simulink model "MdEnChk4s"  (R2018b)
settings: Solver=FixedStepDiscrete  StartTime=0.0  StopTime=10.0  FixedStep=0.01  RelTol=1e-3
undefined symbols (not defined in the file or in its folder): ChkBsyBit, MdAvl, MdEnChk_MdXX_Cal, Req, SetBsyBit, SetEnBit
settings Model: Creator=sn2xws  LastModifiedBy=sn2xws
settings DataIOCC: SaveFormat=StructureWithTime
settings OptimizationCC: DefaultParameterBehavior=Inlined  EnhancedBackFolding=on  PassReuseOutputArgsAs=Individual arguments  ZeroExternalMemoryAtStartup=off  ZeroInternalMemoryAtStartup=off  OptimizeBlockOrder=speed  DifferentSizesBufferReuse=on  OptimizationCustomize=off
settings DebuggingCC: ParameterTunabilityLossMsg=error
settings ModelReferenceCC: ModelReferenceNumInstancesAllowed=Single
settings SFSimCC: MATLABDynamicMemAlloc=off
settings RTWCC: SystemTargetFile=autosar.tlc  GenCodeOnly=on  TemplateMakefile=ert_default_tmf  Description=AUTOSAR  GenerateReport=on  IncludeHyperlinkInReport=on  LaunchReport=on  GenerateTraceInfo=on  GenerateTraceReport=on  GenerateTraceReportSl=on  GenerateTraceReportSf=on  GenerateTraceReportEml=on  GenerateCodeMetricsReport=on
settings CodeAppCC: ForceParamTrailComments=on  IgnoreCustomStorageClasses=off  OperatorAnnotations=on  SimulinkDataObjDesc=on  SFDataObjDesc=on  InsertBlockDesc=on
settings STFCustomTargetCC: TargetLangStandard=C99 (ISO)  MultiwordLength=256  ParMdlRefBuildCompliant=on  CompOptLevelCompliant=on  IncludeMdlTerminateFcn=off  CombineOutputUpdateFcns=on  SuppressErrorStatus=on  ERTCustomFileBanners=on  SupportNonFinite=off  SupportComplex=off  SupportContinuousTime=off  SupportNonInlinedSFcns=off  RemoveResetFunc=on  MATLABClassNameForMDSCustomization=Simulink.SoftwareTarget.ERTCustomization  AutosarCompliant=on  UseToolchainInfoCompliant=on  LookupTableObjectStructAxisOrder=2,1,3,4,...  LUTObjectStructOrderEvenSpacing=Size,Table,Breakpoints  SystemTargetFile=autosar.tlc
settings ERTTargetCC: TargetLangStandard=C99 (ISO)  ConcurrentExecutionCompliant=off  IncludeMdlTerminateFcn=off  SuppressErrorStatus=on  SupportNonFinite=off  SupportComplex=off  ModelStepFunctionPrototypeControlCompliant=off  CPPClassGenCompliant=off  AutosarCompliant=on  LookupTableObjectStructAxisOrder=2,1,3,4,...  LUTObjectStructOrderEvenSpacing=Size,Table,Breakpoints  InlinedParameterPlacement=NonHierarchical  ERTCustomFileTemplate=example_file_process.tlc  ERTFilePackagingFormat=Compact

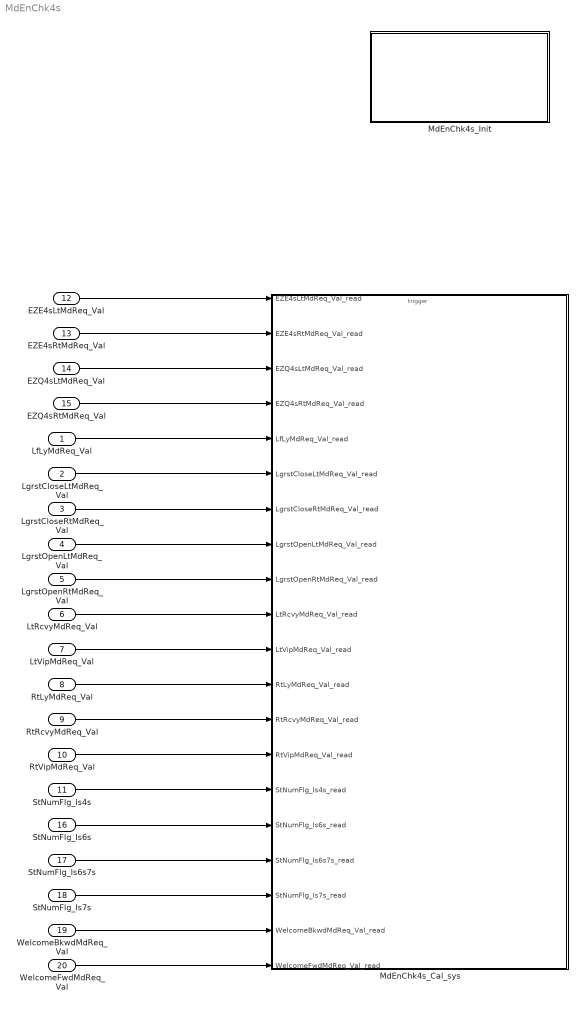
== system MdEnChk4s ==
  LfLyMdReq_Val : Inport  OutDataTypeStr=boolean  PortDimensions=1
  LgrstCloseLtMdReq_Val : Inport  Port=2  OutDataTypeStr=boolean  PortDimensions=1
  LgrstCloseRtMdReq_Val : Inport  Port=3  OutDataTypeStr=boolean  PortDimensions=1
  LgrstOpenLtMdReq_Val : Inport  Port=4  OutDataTypeStr=boolean  PortDimensions=1
  LgrstOpenRtMdReq_Val : Inport  Port=5  OutDataTypeStr=boolean  PortDimensions=1
  LtRcvyMdReq_Val : Inport  Port=6  OutDataTypeStr=boolean  PortDimensions=1
  LtVipMdReq_Val : Inport  Port=7  OutDataTypeStr=boolean  PortDimensions=1
  RtLyMdReq_Val : Inport  Port=8  OutDataTypeStr=boolean  PortDimensions=1
  RtRcvyMdReq_Val : Inport  Port=9  OutDataTypeStr=boolean  PortDimensions=1
  RtVipMdReq_Val : Inport  Port=10  OutDataTypeStr=boolean  PortDimensions=1
  StNumFlg_Is4s : Inport  Port=11  OutDataTypeStr=boolean  PortDimensions=1
  EZE4sLtMdReq_Val : Inport  Port=12  OutDataTypeStr=boolean  PortDimensions=1
  EZE4sRtMdReq_Val : Inport  Port=13  OutDataTypeStr=boolean  PortDimensions=1
  EZQ4sLtMdReq_Val : Inport  Port=14  OutDataTypeStr=boolean  PortDimensions=1
  EZQ4sRtMdReq_Val : Inport  Port=15  OutDataTypeStr=boolean  PortDimensions=1
  StNumFlg_Is6s : Inport  Port=16  OutDataTypeStr=boolean  PortDimensions=1
  StNumFlg_Is6s7s : Inport  Port=17  OutDataTypeStr=boolean  PortDimensions=1
  StNumFlg_Is7s : Inport  Port=18  OutDataTypeStr=boolean  PortDimensions=1
  WelcomeBkwdMdReq_Val : Inport  Port=19  OutDataTypeStr=boolean  PortDimensions=1
  WelcomeFwdMdReq_Val : Inport  Port=20  OutDataTypeStr=boolean  PortDimensions=1
  MdEnChk4s_Cal_sys : Subsystem
  MdEnChk4s_Init : Subsystem
  wires:
  LfLyMdReq_Val/1 -> MdEnChk4s_Cal_sys/5(LfLyMdReq_Val_read)
  LgrstCloseLtMdReq_Val/1 -> MdEnChk4s_Cal_sys/6(LgrstCloseLtMdReq_Val_read)
  LgrstCloseRtMdReq_Val/1 -> MdEnChk4s_Cal_sys/7(LgrstCloseRtMdReq_Val_read)
  LgrstOpenLtMdReq_Val/1 -> MdEnChk4s_Cal_sys/8(LgrstOpenLtMdReq_Val_read)
  LgrstOpenRtMdReq_Val/1 -> MdEnChk4s_Cal_sys/9(LgrstOpenRtMdReq_Val_read)
  LtRcvyMdReq_Val/1 -> MdEnChk4s_Cal_sys/10(LtRcvyMdReq_Val_read)
  LtVipMdReq_Val/1 -> MdEnChk4s_Cal_sys/11(LtVipMdReq_Val_read)
  RtLyMdReq_Val/1 -> MdEnChk4s_Cal_sys/12(RtLyMdReq_Val_read)
  RtRcvyMdReq_Val/1 -> MdEnChk4s_Cal_sys/13(RtRcvyMdReq_Val_read)
  RtVipMdReq_Val/1 -> MdEnChk4s_Cal_sys/14(RtVipMdReq_Val_read)
  StNumFlg_Is4s/1 -> MdEnChk4s_Cal_sys/15(StNumFlg_Is4s_read)
  EZE4sLtMdReq_Val/1 -> MdEnChk4s_Cal_sys/1(EZE4sLtMdReq_Val_read)
  EZE4sRtMdReq_Val/1 -> MdEnChk4s_Cal_sys/2(EZE4sRtMdReq_Val_read)
  EZQ4sLtMdReq_Val/1 -> MdEnChk4s_Cal_sys/3(EZQ4sLtMdReq_Val_read)
  EZQ4sRtMdReq_Val/1 -> MdEnChk4s_Cal_sys/4(EZQ4sRtMdReq_Val_read)
  StNumFlg_Is6s/1 -> MdEnChk4s_Cal_sys/16(StNumFlg_Is6s_read)
  StNumFlg_Is6s7s/1 -> MdEnChk4s_Cal_sys/17(StNumFlg_Is6s7s_read)
  StNumFlg_Is7s/1 -> MdEnChk4s_Cal_sys/18(StNumFlg_Is7s_read)
  WelcomeBkwdMdReq_Val/1 -> MdEnChk4s_Cal_sys/19(WelcomeBkwdMdReq_Val_read)
  WelcomeFwdMdReq_Val/1 -> MdEnChk4s_Cal_sys/20(WelcomeFwdMdReq_Val_read)

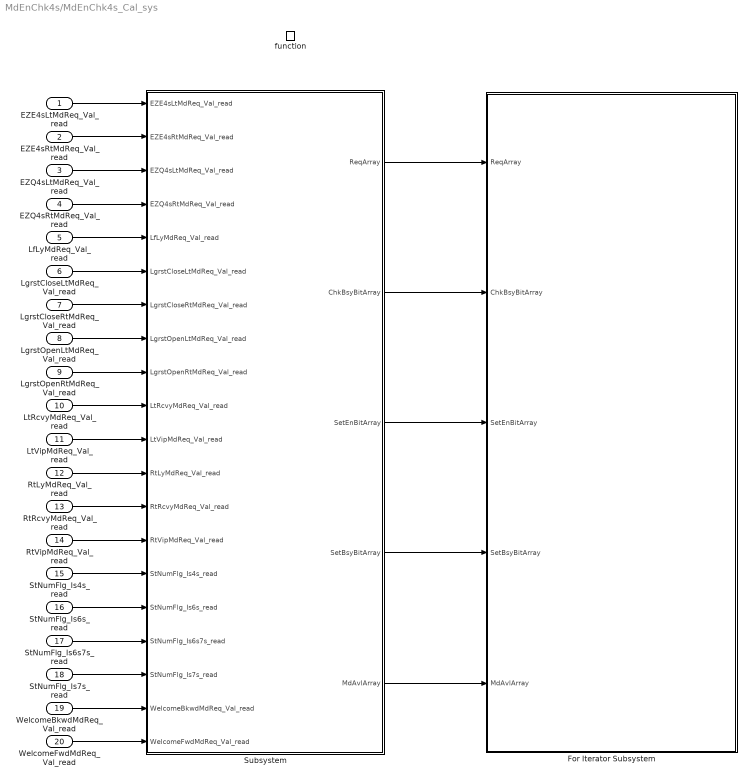
== system MdEnChk4s/MdEnChk4s_Cal_sys ==
  EZE4sLtMdReq_Val_read : Inport
  EZE4sRtMdReq_Val_read : Inport  Port=2
  EZQ4sLtMdReq_Val_read : Inport  Port=3
  EZQ4sRtMdReq_Val_read : Inport  Port=4
  LfLyMdReq_Val_read : Inport  Port=5
  LgrstCloseLtMdReq_Val_read : Inport  Port=6
  LgrstCloseRtMdReq_Val_read : Inport  Port=7
  LgrstOpenLtMdReq_Val_read : Inport  Port=8
  LgrstOpenRtMdReq_Val_read : Inport  Port=9
  LtRcvyMdReq_Val_read : Inport  Port=10
  LtVipMdReq_Val_read : Inport  Port=11
  RtLyMdReq_Val_read : Inport  Port=12
  RtRcvyMdReq_Val_read : Inport  Port=13
  RtVipMdReq_Val_read : Inport  Port=14
  StNumFlg_Is4s_read : Inport  Port=15
  StNumFlg_Is6s_read : Inport  Port=16
  StNumFlg_Is6s7s_read : Inport  Port=17
  StNumFlg_Is7s_read : Inport  Port=18
  WelcomeBkwdMdReq_Val_read : Inport  Port=19
  WelcomeFwdMdReq_Val_read : Inport  Port=20
  function : TriggerPort  TriggerType=function-call  IsSimulinkFunction=on  FunctionName=MdEnChk4s_Cal  VariantControl=(inherit)
  For Iterator Subsystem : Subsystem  TreatAsAtomicUnit=on
  Subsystem : Subsystem
  wires:
  EZE4sLtMdReq_Val_read/1 -> Subsystem/1(EZE4sLtMdReq_Val_read)
  EZE4sRtMdReq_Val_read/1 -> Subsystem/2(EZE4sRtMdReq_Val_read)
  EZQ4sLtMdReq_Val_read/1 -> Subsystem/3(EZQ4sLtMdReq_Val_read)
  EZQ4sRtMdReq_Val_read/1 -> Subsystem/4(EZQ4sRtMdReq_Val_read)
  LfLyMdReq_Val_read/1 -> Subsystem/5(LfLyMdReq_Val_read)
  LgrstCloseLtMdReq_Val_read/1 -> Subsystem/6(LgrstCloseLtMdReq_Val_read)
  LgrstCloseRtMdReq_Val_read/1 -> Subsystem/7(LgrstCloseRtMdReq_Val_read)
  LgrstOpenLtMdReq_Val_read/1 -> Subsystem/8(LgrstOpenLtMdReq_Val_read)
  LgrstOpenRtMdReq_Val_read/1 -> Subsystem/9(LgrstOpenRtMdReq_Val_read)
  LtRcvyMdReq_Val_read/1 -> Subsystem/10(LtRcvyMdReq_Val_read)
  LtVipMdReq_Val_read/1 -> Subsystem/11(LtVipMdReq_Val_read)
  RtLyMdReq_Val_read/1 -> Subsystem/12(RtLyMdReq_Val_read)
  RtRcvyMdReq_Val_read/1 -> Subsystem/13(RtRcvyMdReq_Val_read)
  RtVipMdReq_Val_read/1 -> Subsystem/14(RtVipMdReq_Val_read)
  StNumFlg_Is4s_read/1 -> Subsystem/15(StNumFlg_Is4s_read)
  StNumFlg_Is6s_read/1 -> Subsystem/16(StNumFlg_Is6s_read)
  StNumFlg_Is6s7s_read/1 -> Subsystem/17(StNumFlg_Is6s7s_read)
  StNumFlg_Is7s_read/1 -> Subsystem/18(StNumFlg_Is7s_read)
  WelcomeBkwdMdReq_Val_read/1 -> Subsystem/19(WelcomeBkwdMdReq_Val_read)
  WelcomeFwdMdReq_Val_read/1 -> Subsystem/20(WelcomeFwdMdReq_Val_read)
  Subsystem/1(ReqArray) -> For Iterator Subsystem/1(ReqArray)
  Subsystem/2(ChkBsyBitArray) -> For Iterator Subsystem/2(ChkBsyBitArray)
  Subsystem/3(SetEnBitArray) -> For Iterator Subsystem/3(SetEnBitArray)
  Subsystem/4(SetBsyBitArray) -> For Iterator Subsystem/4(SetBsyBitArray)
  Subsystem/5(MdAvlArray) -> For Iterator Subsystem/5(MdAvlArray)

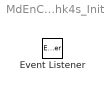
== system MdEnChk4s/MdEnChk4s_Init ==
  Event Listener : EventListener  EventName=reset

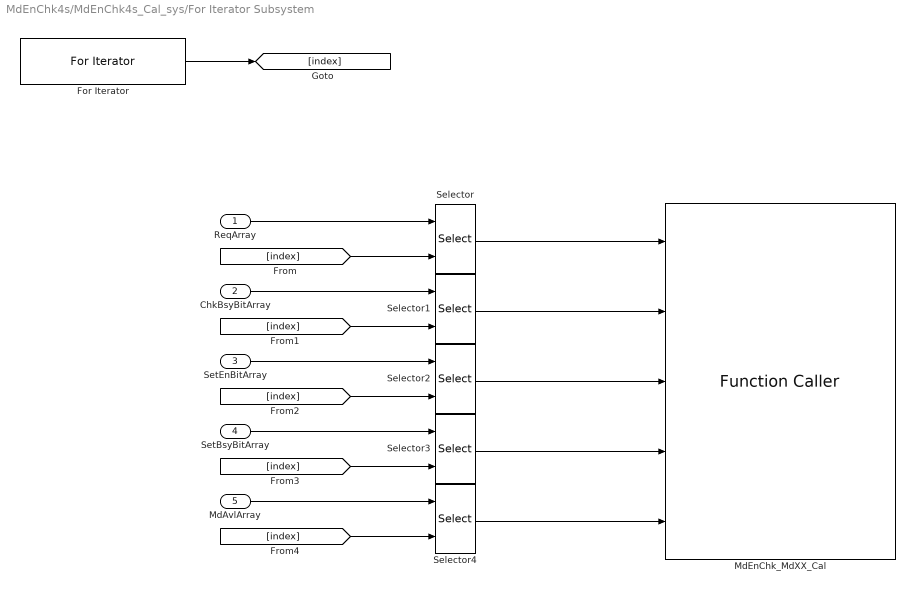
== system MdEnChk4s/MdEnChk4s_Cal_sys/For Iterator Subsystem ==
  ReqArray : Inport
  ChkBsyBitArray : Inport  Port=2
  SetEnBitArray : Inport  Port=3
  SetBsyBitArray : Inport  Port=4
  MdAvlArray : Inport  Port=5
  For Iterator : ForIterator  IterationLimit=16  IndexMode=Zero-based  IterationVariableDataType=int8
  MdEnChk_MdXX_Cal : FunctionCaller  Description=|  FunctionPrototype=MdEnChk_MdXX_Cal(Req,ChkBsyBit,SetEnBit,SetBsyBit,MdAvl)  InputArgumentSpecifications=boolean(true), uint32(1), uint32(1), uint32(1), boolean(true)
      | StNun: 
      | 0 :4s
      | 1:6s
      | 2:7s
      | 3:4sp
  Selector{,1..4} (5 alike) : Selector  IndexMode=Zero-based  InputPortWidth=16  IndexOptions=Index vector (port)  Indices=[1 3]  OutputSizes=1
  wires:
  For Iterator/1 -> [index]
  [index] -> Selector/2
  Selector/1 -> MdEnChk_MdXX_Cal/1
  ReqArray/1 -> Selector/1
  ChkBsyBitArray/1 -> Selector1/1
  [index] -> Selector1/2
  Selector1/1 -> MdEnChk_MdXX_Cal/2
  [index] -> Selector2/2
  SetEnBitArray/1 -> Selector2/1
  Selector2/1 -> MdEnChk_MdXX_Cal/3
  SetBsyBitArray/1 -> Selector3/1
  [index] -> Selector3/2
  Selector3/1 -> MdEnChk_MdXX_Cal/4
  Selector4/1 -> MdEnChk_MdXX_Cal/5
  [index] -> Selector4/2
  MdAvlArray/1 -> Selector4/1

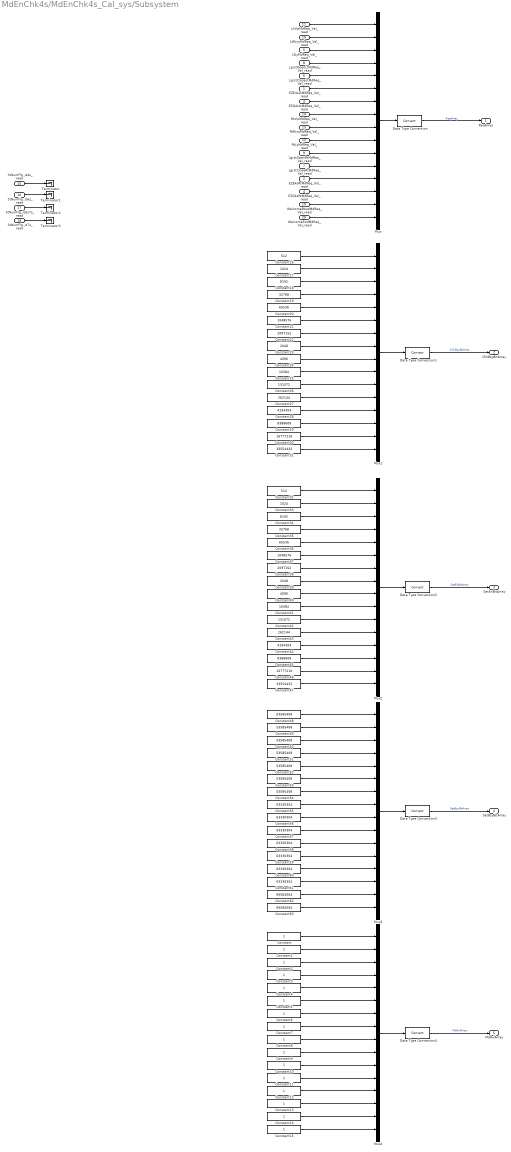
== system MdEnChk4s/MdEnChk4s_Cal_sys/Subsystem ==
  EZE4sLtMdReq_Val_read : Inport
  EZE4sRtMdReq_Val_read : Inport  Port=2
  EZQ4sLtMdReq_Val_read : Inport  Port=3
  EZQ4sRtMdReq_Val_read : Inport  Port=4
  LfLyMdReq_Val_read : Inport  Port=5
  LgrstCloseLtMdReq_Val_read : Inport  Port=6
  LgrstCloseRtMdReq_Val_read : Inport  Port=7
  LgrstOpenLtMdReq_Val_read : Inport  Port=8
  LgrstOpenRtMdReq_Val_read : Inport  Port=9
  LtRcvyMdReq_Val_read : Inport  Port=10
  LtVipMdReq_Val_read : Inport  Port=11
  RtLyMdReq_Val_read : Inport  Port=12
  RtRcvyMdReq_Val_read : Inport  Port=13
  RtVipMdReq_Val_read : Inport  Port=14
  StNumFlg_Is4s_read : Inport  Port=15
  StNumFlg_Is6s_read : Inport  Port=16
  StNumFlg_Is6s7s_read : Inport  Port=17
  StNumFlg_Is7s_read : Inport  Port=18
  WelcomeBkwdMdReq_Val_read : Inport  Port=19
  WelcomeFwdMdReq_Val_read : Inport  Port=20
  Constant{,1..15} (16 alike) : Constant  OutDataTypeStr=boolean
  Constant16 : Constant  Value=512  OutDataTypeStr=uint32
  Constant17 : Constant  Value=1024  OutDataTypeStr=uint32
  Constant18 : Constant  Value=8192  OutDataTypeStr=uint32
  Constant19 : Constant  Value=32768  OutDataTypeStr=uint32
  Constant20 : Constant  Value=65536  OutDataTypeStr=uint32
  Constant21 : Constant  Value=1048576  OutDataTypeStr=uint32
  Constant22 : Constant  Value=2097152  OutDataTypeStr=uint32
  Constant23 : Constant  Value=2048  OutDataTypeStr=uint32
  Constant24 : Constant  Value=4096  OutDataTypeStr=uint32
  Constant25 : Constant  Value=16384  OutDataTypeStr=uint32
  Constant26 : Constant  Value=131072  OutDataTypeStr=uint32
  Constant27 : Constant  Value=262144  OutDataTypeStr=uint32
  Constant28 : Constant  Value=4194304  OutDataTypeStr=uint32
  Constant29 : Constant  Value=8388608  OutDataTypeStr=uint32
  Constant30 : Constant  Value=16777216  OutDataTypeStr=uint32
  Constant31 : Constant  Value=33554432  OutDataTypeStr=uint32
  Constant32 : Constant  Value=512  OutDataTypeStr=uint32
  Constant33 : Constant  Value=1024  OutDataTypeStr=uint32
  Constant34 : Constant  Value=8192  OutDataTypeStr=uint32
  Constant35 : Constant  Value=32768  OutDataTypeStr=uint32
  Constant36 : Constant  Value=65536  OutDataTypeStr=uint32
  Constant37 : Constant  Value=1048576  OutDataTypeStr=uint32
  Constant38 : Constant  Value=2097152  OutDataTypeStr=uint32
  Constant39 : Constant  Value=2048  OutDataTypeStr=uint32
  Constant40 : Constant  Value=4096  OutDataTypeStr=uint32
  Constant41 : Constant  Value=16384  OutDataTypeStr=uint32
  Constant42 : Constant  Value=131072  OutDataTypeStr=uint32
  Constant43 : Constant  Value=262144  OutDataTypeStr=uint32
  Constant44 : Constant  Value=4194304  OutDataTypeStr=uint32
  Constant45 : Constant  Value=8388608  OutDataTypeStr=uint32
  Constant46 : Constant  Value=16777216  OutDataTypeStr=uint32
  Constant47 : Constant  Value=33554432  OutDataTypeStr=uint32
  Constant{48..54} (7 alike) : Constant  Value=53585408  OutDataTypeStr=uint32
  Constant{55..61} (7 alike) : Constant  Value=63330304  OutDataTypeStr=uint32
  Constant62 : Constant  Value=66584064  OutDataTypeStr=uint32
  Constant63 : Constant  Value=66584064  OutDataTypeStr=uint32
  Data Type Conversion{,1..4} (5 alike) : DataTypeConversion
  Mux{,1..4} (5 alike) : Mux  Inputs=16
  Terminator{,1..3} (4 alike) : Terminator
  ReqArray : Outport
  ChkBsyBitArray : Outport  Port=2
  SetEnBitArray : Outport  Port=3
  SetBsyBitArray : Outport  Port=4
  MdAvlArray : Outport  Port=5
  wires:
  LgrstOpenLtMdReq_Val_read/1 -> Mux/4
  LgrstCloseLtMdReq_Val_read/1 -> Mux/5
  EZE4sLtMdReq_Val_read/1 -> Mux/6
  RtRcvyMdReq_Val_read/1 -> Mux/9
  RtLyMdReq_Val_read/1 -> Mux/10
  LgrstOpenRtMdReq_Val_read/1 -> Mux/11
  LgrstCloseRtMdReq_Val_read/1 -> Mux/12
  LtVipMdReq_Val_read/1 -> Mux/1
  LtRcvyMdReq_Val_read/1 -> Mux/2
  LfLyMdReq_Val_read/1 -> Mux/3
  EZQ4sLtMdReq_Val_read/1 -> Mux/7
  RtVipMdReq_Val_read/1 -> Mux/8
  EZE4sRtMdReq_Val_read/1 -> Mux/13
  EZQ4sRtMdReq_Val_read/1 -> Mux/14
  WelcomeBkwdMdReq_Val_read/1 -> Mux/15
  WelcomeFwdMdReq_Val_read/1 -> Mux/16
  Mux/1 -> Data Type Conversion/1
  Data Type Conversion/1 -> ReqArray/1  "ReqArray"
  StNumFlg_Is4s_read/1 -> Terminator/1
  StNumFlg_Is6s_read/1 -> Terminator1/1
  StNumFlg_Is6s7s_read/1 -> Terminator2/1
  StNumFlg_Is7s_read/1 -> Terminator3/1
  Data Type Conversion1/1 -> ChkBsyBitArray/1  "ChkBsyBitArray"
  Mux1/1 -> Data Type Conversion1/1
  Mux2/1 -> Data Type Conversion2/1
  Data Type Conversion2/1 -> SetEnBitArray/1  "SetEnBitArray"
  Data Type Conversion3/1 -> SetBsyBitArray/1  "SetBsyBitArray"
  Mux3/1 -> Data Type Conversion3/1
  Mux4/1 -> Data Type Conversion4/1
  Data Type Conversion4/1 -> MdAvlArray/1  "MdAvlArray"
  Constant/1 -> Mux4/1
  Constant1/1 -> Mux4/2
  Constant2/1 -> Mux4/3
  Constant3/1 -> Mux4/4
  Constant4/1 -> Mux4/5
  Constant5/1 -> Mux4/6
  Constant6/1 -> Mux4/7
  Constant7/1 -> Mux4/8
  Constant8/1 -> Mux4/9
  Constant9/1 -> Mux4/10
  Constant10/1 -> Mux4/11
  Constant11/1 -> Mux4/12
  Constant12/1 -> Mux4/13
  Constant13/1 -> Mux4/14
  Constant14/1 -> Mux4/15
  Constant15/1 -> Mux4/16
  Constant16/1 -> Mux1/1
  Constant17/1 -> Mux1/2
  Constant18/1 -> Mux1/3
  Constant19/1 -> Mux1/4
  Constant20/1 -> Mux1/5
  Constant21/1 -> Mux1/6
  Constant22/1 -> Mux1/7
  Constant23/1 -> Mux1/8
  Constant24/1 -> Mux1/9
  Constant25/1 -> Mux1/10
  Constant26/1 -> Mux1/11
  Constant27/1 -> Mux1/12
  Constant28/1 -> Mux1/13
  Constant29/1 -> Mux1/14
  Constant30/1 -> Mux1/15
  Constant31/1 -> Mux1/16
  Constant47/1 -> Mux2/16
  Constant46/1 -> Mux2/15
  Constant45/1 -> Mux2/14
  Constant44/1 -> Mux2/13
  Constant43/1 -> Mux2/12
  Constant42/1 -> Mux2/11
  Constant41/1 -> Mux2/10
  Constant40/1 -> Mux2/9
  Constant39/1 -> Mux2/8
  Constant38/1 -> Mux2/7
  Constant37/1 -> Mux2/6
  Constant36/1 -> Mux2/5
  Constant35/1 -> Mux2/4
  Constant34/1 -> Mux2/3
  Constant33/1 -> Mux2/2
  Constant32/1 -> Mux2/1
  Constant48/1 -> Mux3/1
  Constant49/1 -> Mux3/2
  Constant50/1 -> Mux3/3
  Constant51/1 -> Mux3/4
  Constant52/1 -> Mux3/5
  Constant53/1 -> Mux3/6
  Constant54/1 -> Mux3/7
  Constant55/1 -> Mux3/8
  Constant56/1 -> Mux3/9
  Constant57/1 -> Mux3/10
  Constant58/1 -> Mux3/11
  Constant59/1 -> Mux3/12
  Constant60/1 -> Mux3/13
  Constant61/1 -> Mux3/14
  Constant62/1 -> Mux3/15
  Constant63/1 -> Mux3/16
